simulink model "sysgen_oversample2x_2samples_per_clock"  (R2016b)
settings: Solver=VariableStepAuto  StartTime=0.0  StopTime=samples_per_channel*number_channels  RelTol=1e-3
PreLoadFcn:
  | setup
undefined symbols (not defined in the file or in its folder): j
libraries: xbsIndex_r4 x355, dspsigops x2, hdlsllib x2
(part 2 of 3)

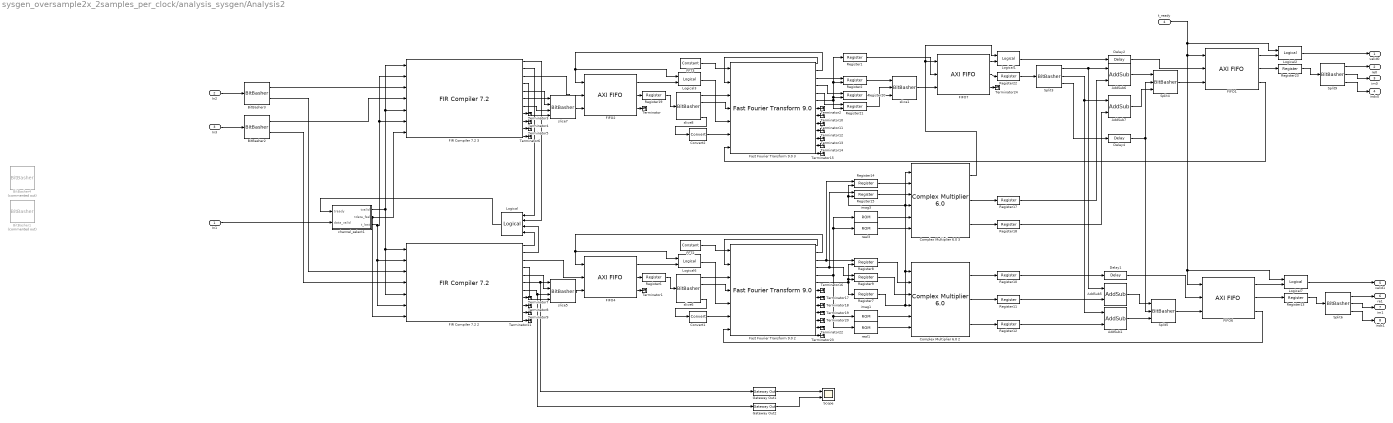
== system sysgen_oversample2x_2samples_per_clock/analysis_sysgen/Analysis2 ==
  In1 : Inport
  In2 : Inport  Port=2
  In3 : Inport  Port=3
  t_ready : Inport  Port=4
  AddSub{1,5..7} (4 alike) : xbsIndex_r4/AddSub  mode=Addition  use_carryin=off  use_carryout=off  en=off  latency=2  precision=Full  arith_type="Signed  (2's comp)"  n_bits=22  bin_pt=16  quantization=Truncate  overflow=Wrap  use_behavioral_HDL=on  hw_selection=Fabric  pipelined=off  dbl_ovrd=off  block_type=addsub
  BitBasher1 : xbsIndex_r4/BitBasher  Commented=on  bitexpr=|  display_expr=off  sr_1=lo  arith_type1="Signed  (2's comp)"  bin_pt1=15  sr_2=hi  arith_type2="Signed  (2's comp)"  bin_pt2=15  sr_3=hi  arith_type3=Unsigned  bin_pt3=0  sr_4=4  arith_type4=Unsigned  bin_pt4=0  dbl_ovrd=off  block_type=bitbasher
      | lo = {in[15:0]}
      | hi = {in[31:16]}
  BitBasher2 : xbsIndex_r4/BitBasher  bitexpr=|  display_expr=off  sr_1=hi  arith_type1="Signed  (2's comp)"  bin_pt1=15  sr_2=lo  arith_type2="Signed  (2's comp)"  bin_pt2=15  sr_3=hi  arith_type3=Unsigned  bin_pt3=0  sr_4=4  arith_type4=Unsigned  bin_pt4=0  dbl_ovrd=off  block_type=bitbasher
      | hi = {in[31:16]}
      | lo = {in[15:0]}
  BitBasher3 : xbsIndex_r4/BitBasher  bitexpr=|  display_expr=off  sr_1=hi  arith_type1="Signed  (2's comp)"  bin_pt1=15  sr_2=lo  arith_type2="Signed  (2's comp)"  bin_pt2=15  sr_3=hi  arith_type3=Unsigned  bin_pt3=0  sr_4=4  arith_type4=Unsigned  bin_pt4=0  dbl_ovrd=off  block_type=bitbasher
      | hi = {in[31:16]}
      | lo = {in[15:0]}
  BitBasher4 : xbsIndex_r4/BitBasher  Commented=on  bitexpr=|  display_expr=off  sr_1=lo  arith_type1="Signed  (2's comp)"  bin_pt1=15  sr_2=hi  arith_type2="Signed  (2's comp)"  bin_pt2=15  sr_3=hi  arith_type3=Unsigned  bin_pt3=0  sr_4=4  arith_type4=Unsigned  bin_pt4=0  dbl_ovrd=off  block_type=bitbasher
      | lo = {in[15:0]}
      | hi = {in[31:16]}
  Complex Multiplier 6.0 2 : xbsIndex_r4/Complex Multiplier 6.0   hasatlast=off  hasatuser=off  atuserwidth=1  hasbtlast=off  hasbtuser=off  btuserwidth=1  multtype=Use_Mults  optimizegoal=Resources  flowcontrol=NonBlocking  outputwidth=24  roundmode=Truncate  hasctrltlast=off  hasctrltuser=off  ctrltuserwidth=1  outtlastbehv=Null  latencyconfig=Automatic  minimumlatency=37  aclken=off  aresetn=off  trim_axipin_name=on  simulation_type=hybrid_sim  simulation_model=sysgen:cmpy_v6_0  data_path_portlist={ 's_axis_a_tdata_real', 's_axis_a_tdata_imag', 's_axis_b_tdata_real', 's_axis_b_tdata_imag', 's_axis_ctrl_tdata_rounding_bit', 'm_axis_dout_tdata_real', 'm_axis_dout_tdata_imag' }  aportwidth=63  bportwidth=63  ip_name=Complex Multiplier  ip_version=6.0  dsptool_ready=true  ipcore_usecache=true  ipcore_useipmodelcache=true  ipcore_verbose=false  ipcore_latency_parameter='minimumlatency'  wrapper_available=true  port_translation_map={ 'aclken' => 'en', 'aresetn' => 'rst'}  block_type=cmpy_v6_0
  Complex Multiplier 6.0 3 : xbsIndex_r4/Complex Multiplier 6.0   hasatlast=off  hasatuser=off  atuserwidth=1  hasbtlast=off  hasbtuser=off  btuserwidth=1  multtype=Use_Mults  optimizegoal=Resources  flowcontrol=NonBlocking  outputwidth=24  roundmode=Truncate  hasctrltlast=off  hasctrltuser=off  ctrltuserwidth=1  outtlastbehv=Null  latencyconfig=Automatic  minimumlatency=37  aclken=off  aresetn=off  trim_axipin_name=on  simulation_type=hybrid_sim  simulation_model=sysgen:cmpy_v6_0  data_path_portlist={ 's_axis_a_tdata_real', 's_axis_a_tdata_imag', 's_axis_b_tdata_real', 's_axis_b_tdata_imag', 's_axis_ctrl_tdata_rounding_bit', 'm_axis_dout_tdata_real', 'm_axis_dout_tdata_imag' }  aportwidth=63  bportwidth=63  ip_name=Complex Multiplier  ip_version=6.0  dsptool_ready=true  ipcore_usecache=true  ipcore_useipmodelcache=true  ipcore_verbose=false  ipcore_latency_parameter='minimumlatency'  wrapper_available=true  port_translation_map={ 'aclken' => 'en', 'aresetn' => 'rst'}  block_type=cmpy_v6_0
  Convert1 : xbsIndex_r4/Convert  gui_display_data_type=Boolean  arith_type=Boolean  n_bits=16  bin_pt=15  float_type=Single  exp_bits=8  fraction_bits=24  quantization=Truncate  overflow=Flag as error  en=off  latency=0  pipeline=off  dbl_ovrd=off  block_type=convert
  Convert2 : xbsIndex_r4/Convert  gui_display_data_type=Boolean  arith_type=Boolean  n_bits=16  bin_pt=15  float_type=Single  exp_bits=8  fraction_bits=24  quantization=Truncate  overflow=Flag as error  en=off  latency=0  pipeline=off  dbl_ovrd=off  block_type=convert
  Delay1 : xbsIndex_r4/Delay  rst=off  infoeditControl=Selection of Reset will increase slice count due to use of real FFs and instead of SRLs  en=off  latency=2  reg_retiming=on  dbl_ovrd=off  block_type=delay
  Delay2 : xbsIndex_r4/Delay  rst=off  infoeditControl=Selection of Reset will increase slice count due to use of real FFs and instead of SRLs  en=off  latency=2  reg_retiming=on  dbl_ovrd=off  block_type=delay
  Delay4 : xbsIndex_r4/Delay  rst=off  infoeditControl=Selection of Reset will increase slice count due to use of real FFs and instead of SRLs  en=off  latency=2  reg_retiming=on  dbl_ovrd=off  block_type=delay
  FFT2 : xbsIndex_r4/Constant  const=1  gui_display_data_type=Fixed-point  arith_type=Unsigned  n_bits=1  bin_pt=0  preci_type=Single  exp_width=8  frac_width=24  explicit_period=off  period=1  equ=P=C  opselect=C  inp2=PCIN>>17  opr=+  inp1=P  carry=CIN  dbl_ovrd=off  block_type=constant
  FFT3 : xbsIndex_r4/Constant  const=1  gui_display_data_type=Fixed-point  arith_type=Unsigned  n_bits=1  bin_pt=0  preci_type=Single  exp_width=8  frac_width=24  explicit_period=off  period=1  equ=P=C  opselect=C  inp2=PCIN>>17  opr=+  inp1=P  carry=CIN  dbl_ovrd=off  block_type=constant
  FIFO{1..2,4,6} (4 alike) : xbsIndex_r4/AXI FIFO  input_depth_axis=16  actual_fifo_depth_label=18  enable_tdata=on  enable_tdest=off  enable_tstrb=off  enable_tready=on  enable_tid=off  enable_tuser=off  enable_tkeep=off  enable_tlast=off  has_aresetn=off  enable_data_counts_axis=off  fifo_implementation_type_axis=Common Clock Distributed RAM  trim_axipin_name=on  programmable_full_type_axis=Full  full_threshold_assert_value_axis=0  programmable_empty_type_axis=Empty  empty_threshold_assert_value_axis=1022  underflow_flag_axi=0  underflow_sense_axi=Active High  overflow_flag_axi=0  overflow_sense_axi=Active High  block_type=axi_fifo
  FIFO7 : xbsIndex_r4/AXI FIFO  input_depth_axis=32  actual_fifo_depth_label=34  enable_tdata=on  enable_tdest=off  enable_tstrb=off  enable_tready=on  enable_tid=off  enable_tuser=off  enable_tkeep=off  enable_tlast=off  has_aresetn=off  enable_data_counts_axis=off  fifo_implementation_type_axis=Common Clock Distributed RAM  trim_axipin_name=on  programmable_full_type_axis=Full  full_threshold_assert_value_axis=0  programmable_empty_type_axis=Empty  empty_threshold_assert_value_axis=1022  underflow_flag_axi=0  underflow_sense_axi=Active High  overflow_flag_axi=0  overflow_sense_axi=Active High  block_type=axi_fifo
  FIR Compiler 7.2 2 : xbsIndex_r4/FIR Compiler 7.2   coefficientvector=analysis_coefficients2  coefficient_sets=8  coefficient_reload=off  filter_type=Single_Rate  rate_change_type=Integer  interpolation_rate=1  decimation_rate=1  zero_pack_factor=1  channel_sequence=Basic  number_channels=8  pattern_list='P4-0,P4-1,P4-2,P4-3,P4-4'  number_paths=2  ratespecification=Output_Sample_Period  sampleperiod=1.00000000  hardwareoversamplingrate=1  coefficient_sign=Signed  quantization=Quantize_Only  coefficient_width=25  bestprecision=on  coefficient_fractional_bits=28  coefficient_structure=Inferred  output_rounding_mode=Convergent_Rounding_to_Even  output_width=19  filter_architecture=Systolic_Multiply_Accumulate  optimization_goal=Area  optimization_list='None'  data_buffer_type=Automatic  coefficient_buffer_type=Automatic  input_buffer_type=Automatic  output_buffer_type=Automatic  preference_for_other_storage=Automatic  multi_column_support=Automatic  columnconfig='16'  inter_column_pipe_length=4  data_has_tlast=Vector_Framing  m_data_has_tready=off  s_data_has_fifo=off  s_data_has_tuser=Not_Required  m_data_has_tuser=Chan_ID_Field  s_config_sync_mode=On_Vector  s_config_method=By_Channel  num_reload_slots=1  has_aclken=off  has_aresetn=off  infoeditControl=ARESETn must be asserted for a minimum of 2 cycles  reset_data_vector=on  trim_axipin_name=on  simulation_type=hybrid_sim  simulation_model=sysgen:xfirv7_2_cmodel  data_path_portlist={ 's_axis_data_tdata', 'm_axis_data_tdata' }  passband_min=0.0  passband_max=0.5  stopband_min=0.5  stopband_max=1.0  filter_selection=1  gui_behaviour='Sysgen_GUI'  data_sign=Signed  data_width=16  data_fractional_bits=0  data_tuser_width=1  wrapper_available=true  ip_wrap_arbitrary_binary_point=true  ip_name=FIR Compiler  ip_version=7.2  dsptool_ready=true  ipcore_usecache=true  ipcore_useipmodelcache=true  port_translation_map={ 'aclken' => 'en', 'aresetn' => 'rst' }  run_core_at_system_period=true  ipcore_xco_need_fpga_part=true  block_type=fir_compiler_v7_2
      settings: infoedit=Maximum Possible : Maximizes oversampling rate. Abstracted input handshake (no s_data_tvalid) and automatic rate propagation.<br>Hardware Oversampling Rate : Specifies oversampling rate relative to the input sample period. Abstracted input handshake (no s_data_tvalid) and automatic rate propagation.<br>Input/Output Sample Period : Specifies absolute oversampling rate. No input handshake abstraction (exposes s_data_tvalid) and no rate propagation.
  FIR Compiler 7.2 3 : xbsIndex_r4/FIR Compiler 7.2   coefficientvector=analysis_coefficients1  coefficient_sets=8  coefficient_reload=off  filter_type=Single_Rate  rate_change_type=Integer  interpolation_rate=1  decimation_rate=1  zero_pack_factor=1  channel_sequence=Basic  number_channels=8  pattern_list='P4-0,P4-1,P4-2,P4-3,P4-4'  number_paths=2  ratespecification=Output_Sample_Period  sampleperiod=1.00000000  hardwareoversamplingrate=1  coefficient_sign=Signed  quantization=Quantize_Only  coefficient_width=25  bestprecision=on  coefficient_fractional_bits=28  coefficient_structure=Inferred  output_rounding_mode=Convergent_Rounding_to_Even  output_width=19  filter_architecture=Systolic_Multiply_Accumulate  optimization_goal=Area  optimization_list='None'  data_buffer_type=Automatic  coefficient_buffer_type=Automatic  input_buffer_type=Automatic  output_buffer_type=Automatic  preference_for_other_storage=Automatic  multi_column_support=Automatic  columnconfig='16'  inter_column_pipe_length=4  data_has_tlast=Vector_Framing  m_data_has_tready=off  s_data_has_fifo=off  s_data_has_tuser=Not_Required  m_data_has_tuser=Chan_ID_Field  s_config_sync_mode=On_Vector  s_config_method=By_Channel  num_reload_slots=1  has_aclken=off  has_aresetn=off  infoeditControl=ARESETn must be asserted for a minimum of 2 cycles  reset_data_vector=on  trim_axipin_name=on  simulation_type=hybrid_sim  simulation_model=sysgen:xfirv7_2_cmodel  data_path_portlist={ 's_axis_data_tdata', 'm_axis_data_tdata' }  passband_min=0.0  passband_max=0.5  stopband_min=0.5  stopband_max=1.0  filter_selection=1  gui_behaviour='Sysgen_GUI'  data_sign=Signed  data_width=16  data_fractional_bits=0  data_tuser_width=1  wrapper_available=true  ip_wrap_arbitrary_binary_point=true  ip_name=FIR Compiler  ip_version=7.2  dsptool_ready=true  ipcore_usecache=true  ipcore_useipmodelcache=true  port_translation_map={ 'aclken' => 'en', 'aresetn' => 'rst' }  run_core_at_system_period=true  ipcore_xco_need_fpga_part=true  block_type=fir_compiler_v7_2
      settings: infoedit=Maximum Possible : Maximizes oversampling rate. Abstracted input handshake (no s_data_tvalid) and automatic rate propagation.<br>Hardware Oversampling Rate : Specifies oversampling rate relative to the input sample period. Abstracted input handshake (no s_data_tvalid) and automatic rate propagation.<br>Input/Output Sample Period : Specifies absolute oversampling rate. No input handshake abstraction (exposes s_data_tvalid) and no rate propagation.
  Fast Fourier Transform 9.0 2 : xbsIndex_r4/Fast Fourier Transform 9.0   transform_length=8  target_clock_frequency=307  target_data_throughput=50  implementation_options=pipelined_streaming_io  run_time_configurable_transform_length=off  phase_factor_width=17  scaling_options=unscaled  rounding_modes=convergent_rounding  aclken=off  aresetn=off  output_ordering=natural_order  cyclic_prefix_insertion=off  throttle_scheme=nonrealtime  xk_index=on  ovflo=off  trim_axipin_name=on  memory_options_data=block_ram  memory_options_phase_factors=block_ram  number_of_stages_using_block_ram_for_data_and_phase_factors=0  memory_options_reorder=block_ram  memory_options_hybrid=off  complex_mult_type=use_mults_resources  butterfly_type=use_xtremedsp_slices  simulation_type=hybrid_sim  simulation_model=sysgen:xfftv9_cmodel  data_path_portlist={ 's_axis_data_tdata', 'm_axis_data_tdata', 'm_axis_status_tdata', 'event_fft_overflow' }  channels=1  input_ordering=natural_order  input_width=16  ip_name=Fast Fourier Transform  ip_version=9.0  dsptool_ready=true  ipcore_usecache=true  ipcore_useipmodelcache=true  wrapper_available=true  port_translation_map={ 'aclken' => 'en', 'aresetn' => 'rst'}  data_format=fixed_point  block_type=xfft_v9_0
  Fast Fourier Transform 9.0 3 : xbsIndex_r4/Fast Fourier Transform 9.0   transform_length=8  target_clock_frequency=307  target_data_throughput=50  implementation_options=pipelined_streaming_io  run_time_configurable_transform_length=off  phase_factor_width=17  scaling_options=unscaled  rounding_modes=convergent_rounding  aclken=off  aresetn=off  output_ordering=natural_order  cyclic_prefix_insertion=off  throttle_scheme=nonrealtime  xk_index=on  ovflo=off  trim_axipin_name=on  memory_options_data=block_ram  memory_options_phase_factors=block_ram  number_of_stages_using_block_ram_for_data_and_phase_factors=0  memory_options_reorder=block_ram  memory_options_hybrid=off  complex_mult_type=use_mults_resources  butterfly_type=use_xtremedsp_slices  simulation_type=hybrid_sim  simulation_model=sysgen:xfftv9_cmodel  data_path_portlist={ 's_axis_data_tdata', 'm_axis_data_tdata', 'm_axis_status_tdata', 'event_fft_overflow' }  channels=1  input_ordering=natural_order  input_width=16  ip_name=Fast Fourier Transform  ip_version=9.0  dsptool_ready=true  ipcore_usecache=true  ipcore_useipmodelcache=true  wrapper_available=true  port_translation_map={ 'aclken' => 'en', 'aresetn' => 'rst'}  data_format=fixed_point  block_type=xfft_v9_0
  Gateway Out1 : xbsIndex_r4/Gateway Out  inherit_from_input=off  hdl_port=off  rows=1  columns=1  UseAsDAC=off  DACChannel='1'  interface=None  automatic_assignment=on  address_offset=hex2dec('00')  intf_name=''  intf_description=''  timing_constraint=None  locs_specified=off  LOCs={}  io_standard={}  block_type=gatewayout
  Gateway Out2 : xbsIndex_r4/Gateway Out  inherit_from_input=off  hdl_port=off  rows=1  columns=1  UseAsDAC=off  DACChannel='1'  interface=None  automatic_assignment=on  address_offset=hex2dec('00')  intf_name=''  intf_description=''  timing_constraint=None  locs_specified=off  LOCs={}  io_standard={}  block_type=gatewayout
  Logical : xbsIndex_r4/Logical  logical_function=AND  inputs=4  en=off  latency=1  precision=Full  arith_type=Unsigned  n_bits=16  bin_pt=0  align_bp=on  dbl_ovrd=off  block_type=logical
  Logical{1..3,6..7} (5 alike) : xbsIndex_r4/Logical  logical_function=AND  inputs=2  en=off  latency=1  precision=Full  arith_type=Unsigned  n_bits=16  bin_pt=0  align_bp=on  dbl_ovrd=off  block_type=logical
  Register{1,6..7,10..13,17..19,22..23} (12 alike) : xbsIndex_r4/Register  init=0  rst=off  en=off  dbl_ovrd=off  block_type=register
  Register{2,8..9,14..15,20..21} (7 alike) : xbsIndex_r4/Register  init=0  rst=off  en=on  dbl_ovrd=off  block_type=register
  Scope : Scope  NumInputPorts=2
  Split3 : xbsIndex_r4/BitBasher  bitexpr=|  display_expr=off  sr_1=im  arith_type1="Signed  (2's comp)"  bin_pt1=17  sr_2=re  arith_type2="Signed  (2's comp)"  bin_pt2=17  sr_3=indx  arith_type3=Unsigned  bin_pt3=0  sr_4=4  arith_type4=Unsigned  bin_pt4=0  dbl_ovrd=off  block_type=bitbasher
      | im={in[43:22]}
      | re={in[21:0]}
      | indx = {in[46:44]}
  Split4 : xbsIndex_r4/BitBasher  bitexpr=out = {9'b0, indx, im, re}  display_expr=off  sr_1=out  arith_type1="Signed  (2's comp)"  bin_pt1=0  sr_2=im  arith_type2="Signed  (2's comp)"  bin_pt2=18  sr_3=3  arith_type3=Unsigned  bin_pt3=0  sr_4=4  arith_type4=Unsigned  bin_pt4=0  dbl_ovrd=off  block_type=bitbasher
  Split5 : xbsIndex_r4/BitBasher  bitexpr=out = {9'b0, indx, im, re}  display_expr=off  sr_1=out  arith_type1="Signed  (2's comp)"  bin_pt1=0  sr_2=im  arith_type2="Signed  (2's comp)"  bin_pt2=18  sr_3=3  arith_type3=Unsigned  bin_pt3=0  sr_4=4  arith_type4=Unsigned  bin_pt4=0  dbl_ovrd=off  block_type=bitbasher
  Split6 : xbsIndex_r4/BitBasher  bitexpr=|  display_expr=off  sr_1=re  arith_type1="Signed  (2's comp)"  bin_pt1=16  sr_2=im  arith_type2="Signed  (2's comp)"  bin_pt2=16  sr_3=indx  arith_type3=Unsigned  bin_pt3=0  sr_4=4  arith_type4=Unsigned  bin_pt4=0  dbl_ovrd=off  block_type=bitbasher
      | re={in[17:0]}
      | im={in[43:26]}
      | indx ={in[52:54]}
  Split9 : xbsIndex_r4/BitBasher  bitexpr=|  display_expr=off  sr_1=re  arith_type1="Signed  (2's comp)"  bin_pt1=16  sr_2=im  arith_type2="Signed  (2's comp)"  bin_pt2=16  sr_3=indx  arith_type3=Unsigned  bin_pt3=0  sr_4=4  arith_type4=Unsigned  bin_pt4=0  dbl_ovrd=off  block_type=bitbasher
      | re={in[17:0]}
      | im={in[43:26]}
      | indx ={in[54:52]}
  Terminator{,1..24} (25 alike) : Terminator
  channel_select1 : Subsystem
  imag1 : xbsIndex_r4/ROM  depth=8  initVector=imag(exp(-j*2*pi*(8:15)/16))  distributed_mem=Block RAM  rst=off  init_reg=0  en=off  latency=1  gui_display_data_type=Fixed-point  arith_type="Signed  (2's comp)"  n_bits=18  bin_pt=16  preci_type=Single  exp_width=8  frac_width=24  optimize=Area  use_rpm=on  dbl_ovrd=off  block_type=sprom
  imag3 : xbsIndex_r4/ROM  depth=8  initVector=imag(exp(-j*2*pi*(0:7)/16))  distributed_mem=Block RAM  rst=off  init_reg=0  en=off  latency=1  gui_display_data_type=Fixed-point  arith_type="Signed  (2's comp)"  n_bits=18  bin_pt=16  preci_type=Single  exp_width=8  frac_width=24  optimize=Area  use_rpm=on  dbl_ovrd=off  block_type=sprom
  real1 : xbsIndex_r4/ROM  depth=8  initVector=real(exp(-j*2*pi*(8:15)/16))  distributed_mem=Block RAM  rst=off  init_reg=0  en=off  latency=1  gui_display_data_type=Fixed-point  arith_type="Signed  (2's comp)"  n_bits=18  bin_pt=16  preci_type=Single  exp_width=8  frac_width=24  optimize=Area  use_rpm=on  dbl_ovrd=off  block_type=sprom
  real3 : xbsIndex_r4/ROM  depth=8  initVector=real(exp(-j*2*pi*(0:7)/16))  distributed_mem=Block RAM  rst=off  init_reg=0  en=off  latency=1  gui_display_data_type=Fixed-point  arith_type="Signed  (2's comp)"  n_bits=18  bin_pt=16  preci_type=Single  exp_width=8  frac_width=24  optimize=Area  use_rpm=on  dbl_ovrd=off  block_type=sprom
  slice1 : xbsIndex_r4/BitBasher  bitexpr="out ={17'b0,  indx, im, re }"  display_expr=off  sr_1=out  arith_type1=Unsigned  bin_pt1=0  sr_2=2  arith_type2="Signed  (2's comp)"  bin_pt2=16  sr_3=3  arith_type3=Unsigned  bin_pt3=0  sr_4=4  arith_type4=Unsigned  bin_pt4=0  dbl_ovrd=off  block_type=bitbasher
  slice5 : xbsIndex_r4/BitBasher  bitexpr=out ={19'b0, tlast, indx, im[20:0], re[20:0] }  display_expr=off  sr_1=out  arith_type1=Unsigned  bin_pt1=0  sr_2=2  arith_type2="Signed  (2's comp)"  bin_pt2=16  sr_3=3  arith_type3=Unsigned  bin_pt3=0  sr_4=4  arith_type4=Unsigned  bin_pt4=0  dbl_ovrd=off  block_type=bitbasher
  slice6 : xbsIndex_r4/BitBasher  bitexpr=|  display_expr=off  sr_1=im_out  arith_type1="Signed  (2's comp)"  bin_pt1=17  sr_2=re_out  arith_type2="Signed  (2's comp)"  bin_pt2=17  sr_3=indx  arith_type3=Unsigned  bin_pt3=0  sr_4=tlast  arith_type4=Unsigned  bin_pt4=0  dbl_ovrd=off  block_type=bitbasher
      | im_out ={ in[39:22] }
      | re_out = { in[18:1] }
      | indx    = { in[44:42] } 
      | tlast     = { in[45] }
  slice7 : xbsIndex_r4/BitBasher  bitexpr=out ={19'b0, tlast, indx, im[20:0], re[20:0] }  display_expr=off  sr_1=out  arith_type1=Unsigned  bin_pt1=0  sr_2=2  arith_type2="Signed  (2's comp)"  bin_pt2=16  sr_3=3  arith_type3=Unsigned  bin_pt3=0  sr_4=4  arith_type4=Unsigned  bin_pt4=0  dbl_ovrd=off  block_type=bitbasher
  slice8 : xbsIndex_r4/BitBasher  bitexpr=|  display_expr=off  sr_1=im_out  arith_type1="Signed  (2's comp)"  bin_pt1=17  sr_2=re_out  arith_type2="Signed  (2's comp)"  bin_pt2=17  sr_3=indx  arith_type3=Unsigned  bin_pt3=0  sr_4=tlast  arith_type4=Unsigned  bin_pt4=0  dbl_ovrd=off  block_type=bitbasher
      | im_out ={ in[39:22] }
      | re_out = { in[18:1] }
      | indx    = { in[44:42] } 
      | tlast     = { in[45] }
  valid0 : Outport
  re0 : Outport  Port=2
  im0 : Outport  Port=3
  indx0 : Outport  Port=4
  valid1 : Outport  Port=5
  re1 : Outport  Port=6
  im1 : Outport  Port=7
  indx1 : Outport  Port=8
  wires:
  FIR Compiler 7.2 2/6 -> slice5/1, Gateway Out1/1
  slice6/1 -> Fast Fourier Transform 9.0 2/3
  Gateway Out2/1 -> Scope/2
  Gateway Out1/1 -> Scope/1
  Fast Fourier Transform 9.0 2/5 -> imag3/1, real3/1, imag1/1, real1/1
  FIFO2/1 -> Logical3/2
  FIFO7/3 -> Terminator24/1
  Fast Fourier Transform 9.0 2/13 -> Terminator23/1
  Fast Fourier Transform 9.0 2/12 -> Terminator22/1
  Fast Fourier Transform 9.0 2/11 -> Terminator20/1
  Fast Fourier Transform 9.0 2/10 -> Terminator19/1
  Fast Fourier Transform 9.0 2/9 -> Terminator18/1
  Fast Fourier Transform 9.0 2/8 -> Terminator17/1
  Fast Fourier Transform 9.0 2/7 -> Terminator16/1
  Fast Fourier Transform 9.0 3/13 -> Terminator15/1
  Fast Fourier Transform 9.0 3/12 -> Terminator14/1
  Fast Fourier Transform 9.0 3/11 -> Terminator13/1
  Fast Fourier Transform 9.0 3/10 -> Terminator12/1
  Fast Fourier Transform 9.0 3/9 -> Terminator11/1
  Fast Fourier Transform 9.0 3/8 -> Terminator10/1
  Fast Fourier Transform 9.0 3/7 -> Terminator2/1
  FIFO4/3 -> Terminator1/1
  FIFO2/3 -> Terminator/1
  Split3/3 -> Delay4/1
  FIFO1/3 -> Fast Fourier Transform 9.0 3/7
  FIFO6/3 -> Fast Fourier Transform 9.0 2/7
  FIFO1/2 -> Register23/1
  FIFO1/1 -> Logical2/2
  Split9/3 -> indx0/1
  Split9/2 -> im0/1
  Split9/1 -> re0/1
  Logical2/1 -> valid0/1
  Register23/1 -> Split9/1
  Delay2/1 -> FIFO1/2
  Split4/1 -> FIFO1/3
  AddSub7/1 -> Split4/3
  AddSub6/1 -> Split4/1
  Delay4/1 -> Split4/2, Split5/2
  Logical1/1 -> Delay2/1
  Register18/1 -> AddSub7/2
  Register17/1 -> AddSub6/2
  Split3/2 -> AddSub7/1, AddSub1/1
  Split3/1 -> AddSub6/1, AddSub5/1
  Register22/1 -> Split3/1
  FIFO7/1 -> Logical1/2
  FIFO7/2 -> Register22/1
  slice1/1 -> FIFO7/3
  Register1/1 -> FIFO7/2
  Register20/1 -> slice1/3
  Register21/1 -> slice1/2
  Register2/1 -> slice1/1
  Fast Fourier Transform 9.0 3/5 -> Register21/1
  Fast Fourier Transform 9.0 3/6 -> Register21/2, Register20/2, Register2/2, Register1/1
  Fast Fourier Transform 9.0 3/4 -> Register20/1
  Fast Fourier Transform 9.0 3/3 -> Register2/1
  BitBasher2/1 -> FIR Compiler 7.2 3/4
  BitBasher3/1 -> FIR Compiler 7.2 3/3
  channel_select1/3(t_last) -> FIR Compiler 7.2 2/2, FIR Compiler 7.2 2/6, FIR Compiler 7.2 3/6, FIR Compiler 7.2 3/2
  Convert2/1 -> Fast Fourier Transform 9.0 3/6
  Fast Fourier Transform 9.0 3/1 -> Fast Fourier Transform 9.0 3/2
  FFT3/1 -> Fast Fourier Transform 9.0 3/1
  slice8/4 -> Convert2/1
  Logical3/1 -> Fast Fourier Transform 9.0 3/5
  slice8/2 -> Fast Fourier Transform 9.0 3/4
  slice8/1 -> Fast Fourier Transform 9.0 3/3
  Register19/1 -> slice8/1
  FIFO2/2 -> Register19/1
  Fast Fourier Transform 9.0 3/2 -> Logical3/1, FIFO2/1
  FIR Compiler 7.2 2/11 -> Terminator21/1
  FIR Compiler 7.2 2/10 -> Terminator9/1
  FIR Compiler 7.2 2/9 -> Terminator8/1
  FIR Compiler 7.2 2/8 -> Terminator7/1
  FIR Compiler 7.2 3/11 -> Terminator6/1
  FIR Compiler 7.2 3/10 -> Terminator5/1
  FIR Compiler 7.2 3/9 -> Terminator4/1
  FIR Compiler 7.2 3/8 -> Terminator3/1
  FIR Compiler 7.2 3/3 -> FIFO2/2
  slice7/1 -> FIFO2/3
  FIR Compiler 7.2 3/4 -> slice7/4
  FIR Compiler 7.2 3/5 -> slice7/2
  FIR Compiler 7.2 3/7 -> slice7/3
  FIR Compiler 7.2 3/6 -> slice7/1
  FIR Compiler 7.2 3/2 -> Logical/1
  FIR Compiler 7.2 3/1 -> Logical/2
  FIR Compiler 7.2 2/2 -> Logical/3
  FIR Compiler 7.2 2/1 -> Logical/4
  Complex Multiplier 6.0 3/3 -> Register18/1
  Complex Multiplier 6.0 3/2 -> Register17/1
  Complex Multiplier 6.0 3/1 -> FIFO7/1, Logical1/1
  Register14/1 -> Complex Multiplier 6.0 3/2
  Register15/1 -> Complex Multiplier 6.0 3/3
  real3/1 -> Complex Multiplier 6.0 3/6
  imag3/1 -> Complex Multiplier 6.0 3/5
  Split6/3 -> indx1/1
  Split6/2 -> im1/1
  Split6/1 -> re1/1
  Logical7/1 -> valid1/1
  Register13/1 -> Split6/1
  FIFO6/2 -> Register13/1
  FIFO6/1 -> Logical7/2
  Delay1/1 -> FIFO6/2
  Split5/1 -> FIFO6/3
  AddSub1/1 -> Split5/3
  AddSub5/1 -> Split5/1
  Register10/1 -> Delay1/1
  Register11/1 -> AddSub5/2
  Register12/1 -> AddSub1/2
  Complex Multiplier 6.0 2/1 -> Register10/1
  Complex Multiplier 6.0 2/2 -> Register11/1
  Complex Multiplier 6.0 2/3 -> Register12/1
  Register7/1 -> Complex Multiplier 6.0 2/4, Complex Multiplier 6.0 2/1, Complex Multiplier 6.0 3/1, Complex Multiplier 6.0 3/4, Register15/2, Register14/2
  Register8/1 -> Complex Multiplier 6.0 2/2
  Register9/1 -> Complex Multiplier 6.0 2/3
  real1/1 -> Complex Multiplier 6.0 2/6
  imag1/1 -> Complex Multiplier 6.0 2/5
  Fast Fourier Transform 9.0 2/6 -> Register7/1, Register9/2, Register8/2
  Fast Fourier Transform 9.0 2/4 -> Register9/1, Register15/1
  Fast Fourier Transform 9.0 2/3 -> Register8/1, Register14/1
  Convert1/1 -> Fast Fourier Transform 9.0 2/6
  Fast Fourier Transform 9.0 2/1 -> Fast Fourier Transform 9.0 2/2
  FFT2/1 -> Fast Fourier Transform 9.0 2/1
  slice6/4 -> Convert1/1
  FIR Compiler 7.2 2/4 -> slice5/4
  Logical6/1 -> Fast Fourier Transform 9.0 2/5
  slice6/2 -> Fast Fourier Transform 9.0 2/4
  Register6/1 -> slice6/1
  FIFO4/2 -> Register6/1
  Fast Fourier Transform 9.0 2/2 -> FIFO4/1, Logical6/1
  FIFO4/1 -> Logical6/2
  FIR Compiler 7.2 2/3 -> FIFO4/2
  slice5/1 -> FIFO4/3
  FIR Compiler 7.2 2/5 -> slice5/2
  FIR Compiler 7.2 2/7 -> slice5/3, Gateway Out2/1
  Logical/1 -> channel_select1/1(tready)
  In1/1 -> channel_select1/2(data_valid)
  BitBasher2/2 -> FIR Compiler 7.2 2/4
  In3/1 -> BitBasher2/1
  BitBasher3/2 -> FIR Compiler 7.2 2/3
  In2/1 -> BitBasher3/1
  channel_select1/1(tvalid) -> FIR Compiler 7.2 2/1, FIR Compiler 7.2 2/5, FIR Compiler 7.2 3/1, FIR Compiler 7.2 3/5
  channel_select1/2(tdata_fsel) -> FIR Compiler 7.2 3/7, FIR Compiler 7.2 2/7
  t_ready/1 -> FIFO6/1, Logical7/1, FIFO1/1, Logical2/1

== system sysgen_oversample2x_2samples_per_clock/analysis_sysgen/Enabled Subsystem ==
  In1 : Inport
  Enable : EnablePort
  Buffer : Buffer  N=8  TreatMby1Signals=One channel  OutputFrames=off
  Out1 : Outport
  wires:
  In1/1 -> Buffer/1
  Buffer/1 -> Out1/1

== system sysgen_oversample2x_2samples_per_clock/analysis_sysgen/Enabled Subsystem2 ==
  In1 : Inport
  Enable : EnablePort
  Buffer : Buffer  N=8  TreatMby1Signals=One channel  OutputFrames=off
  Out1 : Outport
  wires:
  Buffer/1 -> Out1/1
  In1/1 -> Buffer/1

== system sysgen_oversample2x_2samples_per_clock/analysis_sysgen/Enabled Subsystem3 ==
  In1 : Inport
  Enable : EnablePort
  Buffer : Buffer  N=8  TreatMby1Signals=One channel  OutputFrames=off
  Out1 : Outport
  wires:
  In1/1 -> Buffer/1
  Buffer/1 -> Out1/1

== system sysgen_oversample2x_2samples_per_clock/analysis_sysgen/Enabled Subsystem4 ==
  In1 : Inport
  Enable : EnablePort
  Buffer : Buffer  N=8  TreatMby1Signals=One channel  OutputFrames=off
  Out1 : Outport
  wires:
  In1/1 -> Buffer/1
  Buffer/1 -> Out1/1

== system sysgen_oversample2x_2samples_per_clock/analysis_sysgen/Pre-Analysis0 ==
  valid : Inport
  im : Inport  Port=2
  re : Inport  Port=3
  Delay : xbsIndex_r4/Delay  rst=off  infoeditControl=Selection of Reset will increase slice count due to use of real FFs and instead of SRLs  en=off  latency=7  reg_retiming=on  dbl_ovrd=off  block_type=delay
  Delay1 : xbsIndex_r4/Delay  rst=off  infoeditControl=Selection of Reset will increase slice count due to use of real FFs and instead of SRLs  en=off  latency=7  reg_retiming=on  dbl_ovrd=off  block_type=delay
  Delay2 : xbsIndex_r4/Delay  rst=off  infoeditControl=Selection of Reset will increase slice count due to use of real FFs and instead of SRLs  en=off  latency=7  reg_retiming=on  dbl_ovrd=off  block_type=delay
  valid0 : Outport
  im0 : Outport  Port=2
  reo : Outport  Port=3
  wires:
  valid/1 -> Delay/1
  im/1 -> Delay1/1
  re/1 -> Delay2/1
  Delay/1 -> valid0/1
  Delay1/1 -> im0/1
  Delay2/1 -> reo/1

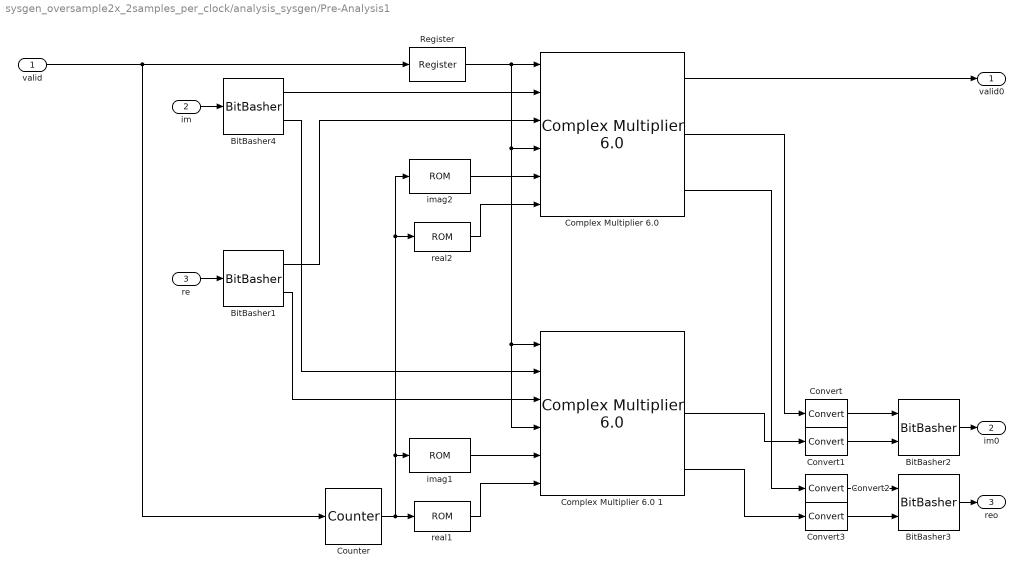
== system sysgen_oversample2x_2samples_per_clock/analysis_sysgen/Pre-Analysis1 ==
  valid : Inport
  im : Inport  Port=2
  re : Inport  Port=3
  BitBasher1 : xbsIndex_r4/BitBasher  bitexpr=|  display_expr=off  sr_1=hi  arith_type1="Signed  (2's comp)"  bin_pt1=15  sr_2=lo  arith_type2="Signed  (2's comp)"  bin_pt2=15  sr_3=hi  arith_type3=Unsigned  bin_pt3=0  sr_4=4  arith_type4=Unsigned  bin_pt4=0  dbl_ovrd=off  block_type=bitbasher
      | hi = {in[31:16]}
      | lo = {in[15:0]}
  BitBasher2 : xbsIndex_r4/BitBasher  bitexpr=out = {hi, lo}  display_expr=off  sr_1=out  arith_type1=Unsigned  bin_pt1=0  sr_2=hi  arith_type2="Signed  (2's comp)"  bin_pt2=15  sr_3=hi  arith_type3=Unsigned  bin_pt3=0  sr_4=4  arith_type4=Unsigned  bin_pt4=0  dbl_ovrd=off  block_type=bitbasher
  BitBasher3 : xbsIndex_r4/BitBasher  bitexpr=out = {hi, lo}  display_expr=off  sr_1=out  arith_type1=Unsigned  bin_pt1=0  sr_2=hi  arith_type2="Signed  (2's comp)"  bin_pt2=15  sr_3=hi  arith_type3=Unsigned  bin_pt3=0  sr_4=4  arith_type4=Unsigned  bin_pt4=0  dbl_ovrd=off  block_type=bitbasher
  BitBasher4 : xbsIndex_r4/BitBasher  bitexpr=|  display_expr=off  sr_1=hi  arith_type1="Signed  (2's comp)"  bin_pt1=15  sr_2=lo  arith_type2="Signed  (2's comp)"  bin_pt2=15  sr_3=hi  arith_type3=Unsigned  bin_pt3=0  sr_4=4  arith_type4=Unsigned  bin_pt4=0  dbl_ovrd=off  block_type=bitbasher
      | hi = {in[31:16]}
      | lo = {in[15:0]}
  "Complex Multiplier 6.0 " : xbsIndex_r4/Complex Multiplier 6.0   hasatlast=off  hasatuser=off  atuserwidth=1  hasbtlast=off  hasbtuser=off  btuserwidth=1  multtype=Use_Mults  optimizegoal=Resources  flowcontrol=NonBlocking  outputwidth=19  roundmode=Truncate  hasctrltlast=off  hasctrltuser=off  ctrltuserwidth=1  outtlastbehv=Null  latencyconfig=Automatic  minimumlatency=37  aclken=off  aresetn=off  trim_axipin_name=on  simulation_type=hybrid_sim  simulation_model=sysgen:cmpy_v6_0  data_path_portlist={ 's_axis_a_tdata_real', 's_axis_a_tdata_imag', 's_axis_b_tdata_real', 's_axis_b_tdata_imag', 's_axis_ctrl_tdata_rounding_bit', 'm_axis_dout_tdata_real', 'm_axis_dout_tdata_imag' }  aportwidth=63  bportwidth=63  ip_name=Complex Multiplier  ip_version=6.0  dsptool_ready=true  ipcore_usecache=true  ipcore_useipmodelcache=true  ipcore_verbose=false  ipcore_latency_parameter='minimumlatency'  wrapper_available=true  port_translation_map={ 'aclken' => 'en', 'aresetn' => 'rst'}  block_type=cmpy_v6_0
  Complex Multiplier 6.0 1 : xbsIndex_r4/Complex Multiplier 6.0   hasatlast=off  hasatuser=off  atuserwidth=1  hasbtlast=off  hasbtuser=off  btuserwidth=1  multtype=Use_Mults  optimizegoal=Resources  flowcontrol=NonBlocking  outputwidth=19  roundmode=Truncate  hasctrltlast=off  hasctrltuser=off  ctrltuserwidth=1  outtlastbehv=Null  latencyconfig=Automatic  minimumlatency=37  aclken=off  aresetn=off  trim_axipin_name=on  simulation_type=hybrid_sim  simulation_model=sysgen:cmpy_v6_0  data_path_portlist={ 's_axis_a_tdata_real', 's_axis_a_tdata_imag', 's_axis_b_tdata_real', 's_axis_b_tdata_imag', 's_axis_ctrl_tdata_rounding_bit', 'm_axis_dout_tdata_real', 'm_axis_dout_tdata_imag' }  aportwidth=63  bportwidth=63  ip_name=Complex Multiplier  ip_version=6.0  dsptool_ready=true  ipcore_usecache=true  ipcore_useipmodelcache=true  ipcore_verbose=false  ipcore_latency_parameter='minimumlatency'  wrapper_available=true  port_translation_map={ 'aclken' => 'en', 'aresetn' => 'rst'}  block_type=cmpy_v6_0
  Convert{,1..3} (4 alike) : xbsIndex_r4/Convert  gui_display_data_type=Fixed-point  arith_type="Signed  (2's comp)"  n_bits=16  bin_pt=15  float_type=Single  exp_bits=8  fraction_bits=24  quantization=Truncate  overflow=Flag as error  en=off  latency=0  pipeline=off  dbl_ovrd=off  block_type=convert
  Counter : xbsIndex_r4/Counter  cnt_type=Free Running  cnt_to=Inf  operation=Up  start_count=0  cnt_by_val=1  arith_type=Unsigned  n_bits=4  bin_pt=0  load_pin=off  rst=off  en=on  explicit_period=on  period=2  use_behavioral_HDL=off  implementation=Fabric  dbl_ovrd=off  block_type=counter
  Register : xbsIndex_r4/Register  init=0  rst=off  en=off  dbl_ovrd=off  block_type=register
  imag1 : xbsIndex_r4/ROM  depth=16  initVector=imag(exp(-j*2*pi*(1:2:31)/32))  distributed_mem=Block RAM  rst=off  init_reg=0  en=off  latency=1  gui_display_data_type=Fixed-point  arith_type="Signed  (2's comp)"  n_bits=18  bin_pt=16  preci_type=Single  exp_width=8  frac_width=24  optimize=Area  use_rpm=on  dbl_ovrd=off  block_type=sprom
  imag2 : xbsIndex_r4/ROM  depth=16  initVector=imag(exp(-j*2*pi*(0:2:31)/32))  distributed_mem=Block RAM  rst=off  init_reg=0  en=off  latency=1  gui_display_data_type=Fixed-point  arith_type="Signed  (2's comp)"  n_bits=18  bin_pt=16  preci_type=Single  exp_width=8  frac_width=24  optimize=Area  use_rpm=on  dbl_ovrd=off  block_type=sprom
  real1 : xbsIndex_r4/ROM  depth=16  initVector=real(exp(-j*2*pi*(1:2:31)/32))  distributed_mem=Block RAM  rst=off  init_reg=0  en=off  latency=1  gui_display_data_type=Fixed-point  arith_type="Signed  (2's comp)"  n_bits=18  bin_pt=16  preci_type=Single  exp_width=8  frac_width=24  optimize=Area  use_rpm=on  dbl_ovrd=off  block_type=sprom
  real2 : xbsIndex_r4/ROM  depth=16  initVector=real(exp(-j*2*pi*(0:2:31)/32))  distributed_mem=Block RAM  rst=off  init_reg=0  en=off  latency=1  gui_display_data_type=Fixed-point  arith_type="Signed  (2's comp)"  n_bits=18  bin_pt=16  preci_type=Single  exp_width=8  frac_width=24  optimize=Area  use_rpm=on  dbl_ovrd=off  block_type=sprom
  valid0 : Outport
  im0 : Outport  Port=2
  reo : Outport  Port=3
  wires:
  im/1 -> BitBasher4/1
  re/1 -> BitBasher1/1
  real2/1 -> "Complex Multiplier 6.0 "/6
  imag2/1 -> "Complex Multiplier 6.0 "/5
  BitBasher4/1 -> "Complex Multiplier 6.0 "/2
  real1/1 -> Complex Multiplier 6.0 1/6
  imag1/1 -> Complex Multiplier 6.0 1/5
  BitBasher4/2 -> Complex Multiplier 6.0 1/2
  BitBasher1/2 -> Complex Multiplier 6.0 1/3
  Counter/1 -> imag2/1, real2/1, imag1/1, real1/1
  BitBasher2/1 -> im0/1
  BitBasher3/1 -> reo/1
  valid/1 -> Register/1, Counter/1
  Convert/1 -> BitBasher2/1
  Convert2/1 -> BitBasher3/1
  Convert3/1 -> BitBasher3/2
  Register/1 -> "Complex Multiplier 6.0 "/4, Complex Multiplier 6.0 1/1, Complex Multiplier 6.0 1/4, "Complex Multiplier 6.0 "/1
  "Complex Multiplier 6.0 "/1 -> valid0/1
  Convert1/1 -> BitBasher2/2
  BitBasher1/1 -> "Complex Multiplier 6.0 "/3
  Complex Multiplier 6.0 1/2 -> Convert1/1
  Complex Multiplier 6.0 1/3 -> Convert3/1
  "Complex Multiplier 6.0 "/2 -> Convert/1
  "Complex Multiplier 6.0 "/3 -> Convert2/1

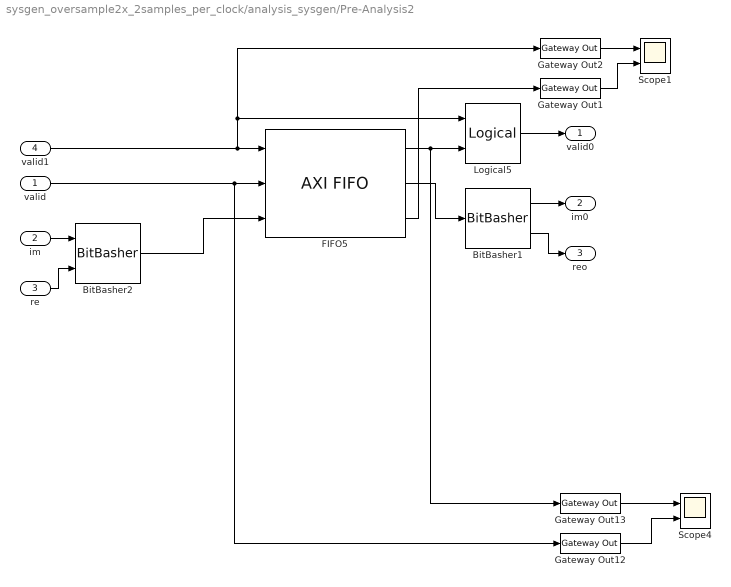
== system sysgen_oversample2x_2samples_per_clock/analysis_sysgen/Pre-Analysis2 ==
  valid : Inport
  im : Inport  Port=2
  re : Inport  Port=3
  valid1 : Inport  Port=4
  BitBasher1 : xbsIndex_r4/BitBasher  bitexpr=|  display_expr=off  sr_1=im  arith_type1=Unsigned  bin_pt1=0  sr_2=re  arith_type2=Unsigned  bin_pt2=0  sr_3=hi  arith_type3=Unsigned  bin_pt3=0  sr_4=4  arith_type4=Unsigned  bin_pt4=0  dbl_ovrd=off  block_type=bitbasher
      | im = {in[63:32]}
      | re = {in[31:0]}
  BitBasher2 : xbsIndex_r4/BitBasher  bitexpr=out = {im, re}  display_expr=off  sr_1=out  arith_type1=Unsigned  bin_pt1=0  sr_2=hi  arith_type2="Signed  (2's comp)"  bin_pt2=15  sr_3=hi  arith_type3=Unsigned  bin_pt3=0  sr_4=4  arith_type4=Unsigned  bin_pt4=0  dbl_ovrd=off  block_type=bitbasher
  FIFO5 : xbsIndex_r4/AXI FIFO  input_depth_axis=16  actual_fifo_depth_label=18  enable_tdata=on  enable_tdest=off  enable_tstrb=off  enable_tready=on  enable_tid=off  enable_tuser=off  enable_tkeep=off  enable_tlast=off  has_aresetn=off  enable_data_counts_axis=off  fifo_implementation_type_axis=Common Clock Distributed RAM  trim_axipin_name=on  programmable_full_type_axis=Full  full_threshold_assert_value_axis=0  programmable_empty_type_axis=Empty  empty_threshold_assert_value_axis=1022  underflow_flag_axi=0  underflow_sense_axi=Active High  overflow_flag_axi=0  overflow_sense_axi=Active High  block_type=axi_fifo
  Gateway Out{1..2,12..13} (4 alike) : xbsIndex_r4/Gateway Out  inherit_from_input=off  hdl_port=off  rows=1  columns=1  UseAsDAC=off  DACChannel='1'  interface=None  automatic_assignment=on  address_offset=hex2dec('00')  intf_name=''  intf_description=''  timing_constraint=None  locs_specified=off  LOCs={}  io_standard={}  block_type=gatewayout
  Logical5 : xbsIndex_r4/Logical  logical_function=AND  inputs=2  en=off  latency=0  precision=Full  arith_type=Unsigned  n_bits=16  bin_pt=0  align_bp=on  dbl_ovrd=off  block_type=logical
  Scope1 : Scope  NumInputPorts=2
  Scope4 : Scope  NumInputPorts=2
  valid0 : Outport
  im0 : Outport  Port=2
  reo : Outport  Port=3
  wires:
  Gateway Out12/1 -> Scope4/2
  Gateway Out13/1 -> Scope4/1
  FIFO5/2 -> BitBasher1/1
  BitBasher1/2 -> reo/1
  BitBasher1/1 -> im0/1
  Logical5/1 -> valid0/1
  FIFO5/1 -> Logical5/2, Gateway Out13/1
  BitBasher2/1 -> FIFO5/3
  re/1 -> BitBasher2/2
  im/1 -> BitBasher2/1
  valid/1 -> FIFO5/2, Gateway Out12/1
  FIFO5/3 -> Gateway Out1/1
  Gateway Out2/1 -> Scope1/1
  Gateway Out1/1 -> Scope1/2
  valid1/1 -> FIFO5/1, Gateway Out2/1, Logical5/1

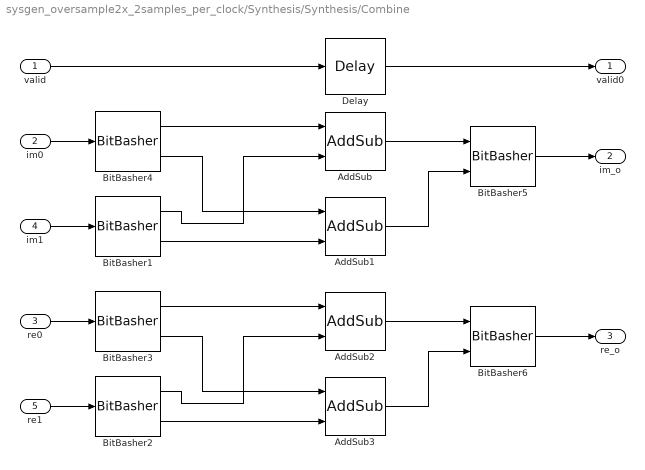
== system sysgen_oversample2x_2samples_per_clock/Synthesis/Synthesis/Combine ==
  valid : Inport
  im0 : Inport  Port=2
  re0 : Inport  Port=3
  im1 : Inport  Port=4
  re1 : Inport  Port=5
  AddSub{,1..3} (4 alike) : xbsIndex_r4/AddSub  mode=Subtraction  use_carryin=off  use_carryout=off  en=off  latency=2  precision=User Defined  arith_type="Signed  (2's comp)"  n_bits=16  bin_pt=15  quantization=Truncate  overflow=Saturate  use_behavioral_HDL=on  hw_selection=Fabric  pipelined=off  dbl_ovrd=off  block_type=addsub
  BitBasher1 : xbsIndex_r4/BitBasher  bitexpr=|  display_expr=off  sr_1=hi  arith_type1="Signed  (2's comp)"  bin_pt1=15  sr_2=lo  arith_type2="Signed  (2's comp)"  bin_pt2=15  sr_3=hi  arith_type3=Unsigned  bin_pt3=0  sr_4=4  arith_type4=Unsigned  bin_pt4=0  dbl_ovrd=off  block_type=bitbasher
      | hi = {in[31:16]}
      | lo = {in[15:0]}
  BitBasher2 : xbsIndex_r4/BitBasher  bitexpr=|  display_expr=off  sr_1=hi  arith_type1="Signed  (2's comp)"  bin_pt1=15  sr_2=lo  arith_type2="Signed  (2's comp)"  bin_pt2=15  sr_3=hi  arith_type3=Unsigned  bin_pt3=0  sr_4=4  arith_type4=Unsigned  bin_pt4=0  dbl_ovrd=off  block_type=bitbasher
      | hi = {in[31:16]}
      | lo = {in[15:0]}
  BitBasher3 : xbsIndex_r4/BitBasher  bitexpr=|  display_expr=off  sr_1=hi  arith_type1="Signed  (2's comp)"  bin_pt1=15  sr_2=lo  arith_type2="Signed  (2's comp)"  bin_pt2=15  sr_3=hi  arith_type3=Unsigned  bin_pt3=0  sr_4=4  arith_type4=Unsigned  bin_pt4=0  dbl_ovrd=off  block_type=bitbasher
      | hi = {in[31:16]}
      | lo = {in[15:0]}
  BitBasher4 : xbsIndex_r4/BitBasher  bitexpr=|  display_expr=off  sr_1=hi  arith_type1="Signed  (2's comp)"  bin_pt1=15  sr_2=lo  arith_type2="Signed  (2's comp)"  bin_pt2=15  sr_3=hi  arith_type3=Unsigned  bin_pt3=0  sr_4=4  arith_type4=Unsigned  bin_pt4=0  dbl_ovrd=off  block_type=bitbasher
      | hi = {in[31:16]}
      | lo = {in[15:0]}
  BitBasher5 : xbsIndex_r4/BitBasher  bitexpr=out = {hi, lo}  display_expr=off  sr_1=out  arith_type1=Unsigned  bin_pt1=0  sr_2=hi  arith_type2="Signed  (2's comp)"  bin_pt2=15  sr_3=hi  arith_type3=Unsigned  bin_pt3=0  sr_4=4  arith_type4=Unsigned  bin_pt4=0  dbl_ovrd=off  block_type=bitbasher
  BitBasher6 : xbsIndex_r4/BitBasher  bitexpr=out = {hi, lo}  display_expr=off  sr_1=out  arith_type1=Unsigned  bin_pt1=0  sr_2=hi  arith_type2="Signed  (2's comp)"  bin_pt2=15  sr_3=hi  arith_type3=Unsigned  bin_pt3=0  sr_4=4  arith_type4=Unsigned  bin_pt4=0  dbl_ovrd=off  block_type=bitbasher
  Delay : xbsIndex_r4/Delay  rst=off  infoeditControl=Selection of Reset will increase slice count due to use of real FFs and instead of SRLs  en=off  latency=2  reg_retiming=on  dbl_ovrd=off  block_type=delay
  valid0 : Outport
  im_o : Outport  Port=2
  re_o : Outport  Port=3
  wires:
  im1/1 -> BitBasher1/1
  im0/1 -> BitBasher4/1
  valid/1 -> Delay/1
  BitBasher4/1 -> AddSub/1
  BitBasher1/1 -> AddSub/2
  BitBasher4/2 -> AddSub1/1
  BitBasher1/2 -> AddSub1/2
  re1/1 -> BitBasher2/1
  re0/1 -> BitBasher3/1
  BitBasher3/1 -> AddSub2/1
  BitBasher2/1 -> AddSub2/2
  BitBasher3/2 -> AddSub3/1
  BitBasher2/2 -> AddSub3/2
  Delay/1 -> valid0/1
  AddSub/1 -> BitBasher5/1
  AddSub1/1 -> BitBasher5/2
  AddSub2/1 -> BitBasher6/1
  AddSub3/1 -> BitBasher6/2
  BitBasher6/1 -> re_o/1
  BitBasher5/1 -> im_o/1

== system sysgen_oversample2x_2samples_per_clock/Synthesis/Synthesis/Post_synthesis0 ==
  valid : Inport
  im : Inport  Port=2
  re : Inport  Port=3
  Delay : xbsIndex_r4/Delay  rst=off  infoeditControl=Selection of Reset will increase slice count due to use of real FFs and instead of SRLs  en=off  latency=7  reg_retiming=on  dbl_ovrd=off  block_type=delay
  Delay1 : xbsIndex_r4/Delay  rst=off  infoeditControl=Selection of Reset will increase slice count due to use of real FFs and instead of SRLs  en=off  latency=7  reg_retiming=on  dbl_ovrd=off  block_type=delay
  Delay2 : xbsIndex_r4/Delay  rst=off  infoeditControl=Selection of Reset will increase slice count due to use of real FFs and instead of SRLs  en=off  latency=7  reg_retiming=on  dbl_ovrd=off  block_type=delay
  valid0 : Outport
  im0 : Outport  Port=2
  reo : Outport  Port=3
  wires:
  valid/1 -> Delay/1
  im/1 -> Delay1/1
  re/1 -> Delay2/1
  Delay/1 -> valid0/1
  Delay1/1 -> im0/1
  Delay2/1 -> reo/1

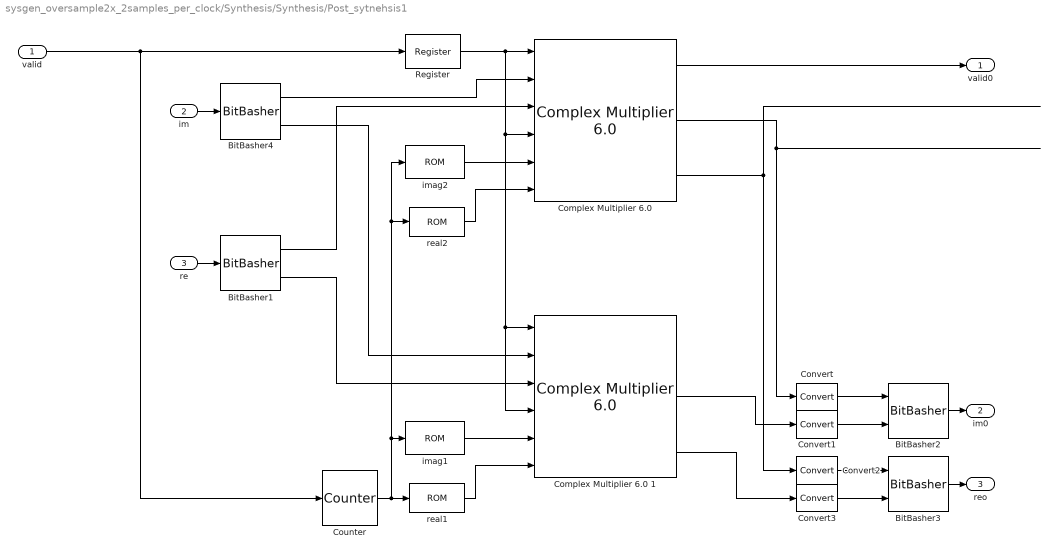
== system sysgen_oversample2x_2samples_per_clock/Synthesis/Synthesis/Post_sytnehsis1 ==
  valid : Inport
  im : Inport  Port=2
  re : Inport  Port=3
  BitBasher1 : xbsIndex_r4/BitBasher  bitexpr=|  display_expr=off  sr_1=hi  arith_type1="Signed  (2's comp)"  bin_pt1=15  sr_2=lo  arith_type2="Signed  (2's comp)"  bin_pt2=15  sr_3=hi  arith_type3=Unsigned  bin_pt3=0  sr_4=4  arith_type4=Unsigned  bin_pt4=0  dbl_ovrd=off  block_type=bitbasher
      | hi = {in[31:16]}
      | lo = {in[15:0]}
  BitBasher2 : xbsIndex_r4/BitBasher  bitexpr=out = {hi, lo}  display_expr=off  sr_1=out  arith_type1=Unsigned  bin_pt1=0  sr_2=hi  arith_type2="Signed  (2's comp)"  bin_pt2=15  sr_3=hi  arith_type3=Unsigned  bin_pt3=0  sr_4=4  arith_type4=Unsigned  bin_pt4=0  dbl_ovrd=off  block_type=bitbasher
  BitBasher3 : xbsIndex_r4/BitBasher  bitexpr=out = {hi, lo}  display_expr=off  sr_1=out  arith_type1=Unsigned  bin_pt1=0  sr_2=hi  arith_type2="Signed  (2's comp)"  bin_pt2=15  sr_3=hi  arith_type3=Unsigned  bin_pt3=0  sr_4=4  arith_type4=Unsigned  bin_pt4=0  dbl_ovrd=off  block_type=bitbasher
  BitBasher4 : xbsIndex_r4/BitBasher  bitexpr=|  display_expr=off  sr_1=hi  arith_type1="Signed  (2's comp)"  bin_pt1=15  sr_2=lo  arith_type2="Signed  (2's comp)"  bin_pt2=15  sr_3=hi  arith_type3=Unsigned  bin_pt3=0  sr_4=4  arith_type4=Unsigned  bin_pt4=0  dbl_ovrd=off  block_type=bitbasher
      | hi = {in[31:16]}
      | lo = {in[15:0]}
  "Complex Multiplier 6.0 " : xbsIndex_r4/Complex Multiplier 6.0   hasatlast=off  hasatuser=off  atuserwidth=1  hasbtlast=off  hasbtuser=off  btuserwidth=1  multtype=Use_Mults  optimizegoal=Resources  flowcontrol=NonBlocking  outputwidth=19  roundmode=Truncate  hasctrltlast=off  hasctrltuser=off  ctrltuserwidth=1  outtlastbehv=Null  latencyconfig=Automatic  minimumlatency=37  aclken=off  aresetn=off  trim_axipin_name=on  simulation_type=hybrid_sim  simulation_model=sysgen:cmpy_v6_0  data_path_portlist={ 's_axis_a_tdata_real', 's_axis_a_tdata_imag', 's_axis_b_tdata_real', 's_axis_b_tdata_imag', 's_axis_ctrl_tdata_rounding_bit', 'm_axis_dout_tdata_real', 'm_axis_dout_tdata_imag' }  aportwidth=63  bportwidth=63  ip_name=Complex Multiplier  ip_version=6.0  dsptool_ready=true  ipcore_usecache=true  ipcore_useipmodelcache=true  ipcore_verbose=false  ipcore_latency_parameter='minimumlatency'  wrapper_available=true  port_translation_map={ 'aclken' => 'en', 'aresetn' => 'rst'}  block_type=cmpy_v6_0
  Complex Multiplier 6.0 1 : xbsIndex_r4/Complex Multiplier 6.0   hasatlast=off  hasatuser=off  atuserwidth=1  hasbtlast=off  hasbtuser=off  btuserwidth=1  multtype=Use_Mults  optimizegoal=Resources  flowcontrol=NonBlocking  outputwidth=19  roundmode=Truncate  hasctrltlast=off  hasctrltuser=off  ctrltuserwidth=1  outtlastbehv=Null  latencyconfig=Automatic  minimumlatency=37  aclken=off  aresetn=off  trim_axipin_name=on  simulation_type=hybrid_sim  simulation_model=sysgen:cmpy_v6_0  data_path_portlist={ 's_axis_a_tdata_real', 's_axis_a_tdata_imag', 's_axis_b_tdata_real', 's_axis_b_tdata_imag', 's_axis_ctrl_tdata_rounding_bit', 'm_axis_dout_tdata_real', 'm_axis_dout_tdata_imag' }  aportwidth=63  bportwidth=63  ip_name=Complex Multiplier  ip_version=6.0  dsptool_ready=true  ipcore_usecache=true  ipcore_useipmodelcache=true  ipcore_verbose=false  ipcore_latency_parameter='minimumlatency'  wrapper_available=true  port_translation_map={ 'aclken' => 'en', 'aresetn' => 'rst'}  block_type=cmpy_v6_0
  Convert{,1..3} (4 alike) : xbsIndex_r4/Convert  gui_display_data_type=Fixed-point  arith_type="Signed  (2's comp)"  n_bits=16  bin_pt=15  float_type=Single  exp_bits=8  fraction_bits=24  quantization=Truncate  overflow=Flag as error  en=off  latency=0  pipeline=off  dbl_ovrd=off  block_type=convert
  Counter : xbsIndex_r4/Counter  cnt_type=Free Running  cnt_to=Inf  operation=Up  start_count=0  cnt_by_val=1  arith_type=Unsigned  n_bits=4  bin_pt=0  load_pin=off  rst=off  en=on  explicit_period=on  period=2  use_behavioral_HDL=off  implementation=Fabric  dbl_ovrd=off  block_type=counter
  Register : xbsIndex_r4/Register  init=0  rst=off  en=off  dbl_ovrd=off  block_type=register
  imag1 : xbsIndex_r4/ROM  depth=16  initVector=imag(exp(j*2*pi*(1:2:31)/32))  distributed_mem=Block RAM  rst=off  init_reg=0  en=off  latency=1  gui_display_data_type=Fixed-point  arith_type="Signed  (2's comp)"  n_bits=18  bin_pt=16  preci_type=Single  exp_width=8  frac_width=24  optimize=Area  use_rpm=on  dbl_ovrd=off  block_type=sprom
  imag2 : xbsIndex_r4/ROM  depth=16  initVector=imag(exp(j*2*pi*(0:2:31)/32))  distributed_mem=Block RAM  rst=off  init_reg=0  en=off  latency=1  gui_display_data_type=Fixed-point  arith_type="Signed  (2's comp)"  n_bits=18  bin_pt=16  preci_type=Single  exp_width=8  frac_width=24  optimize=Area  use_rpm=on  dbl_ovrd=off  block_type=sprom
  real1 : xbsIndex_r4/ROM  depth=16  initVector=real(exp(j*2*pi*(1:2:31)/32))  distributed_mem=Block RAM  rst=off  init_reg=0  en=off  latency=1  gui_display_data_type=Fixed-point  arith_type="Signed  (2's comp)"  n_bits=18  bin_pt=16  preci_type=Single  exp_width=8  frac_width=24  optimize=Area  use_rpm=on  dbl_ovrd=off  block_type=sprom
  real2 : xbsIndex_r4/ROM  depth=16  initVector=real(exp(j*2*pi*(0:2:31)/32))  distributed_mem=Block RAM  rst=off  init_reg=0  en=off  latency=1  gui_display_data_type=Fixed-point  arith_type="Signed  (2's comp)"  n_bits=18  bin_pt=16  preci_type=Single  exp_width=8  frac_width=24  optimize=Area  use_rpm=on  dbl_ovrd=off  block_type=sprom
  valid0 : Outport
  im0 : Outport  Port=2
  reo : Outport  Port=3
  wires:
  im/1 -> BitBasher4/1
  re/1 -> BitBasher1/1
  real2/1 -> "Complex Multiplier 6.0 "/6
  imag2/1 -> "Complex Multiplier 6.0 "/5
  real1/1 -> Complex Multiplier 6.0 1/6
  imag1/1 -> Complex Multiplier 6.0 1/5
  Counter/1 -> imag2/1, real2/1, imag1/1, real1/1
  BitBasher2/1 -> im0/1
  BitBasher3/1 -> reo/1
  valid/1 -> Register/1, Counter/1
  Convert/1 -> BitBasher2/1
  Convert2/1 -> BitBasher3/1
  Convert3/1 -> BitBasher3/2
  Register/1 -> "Complex Multiplier 6.0 "/4, Complex Multiplier 6.0 1/1, Complex Multiplier 6.0 1/4, "Complex Multiplier 6.0 "/1
  "Complex Multiplier 6.0 "/1 -> valid0/1
  Convert1/1 -> BitBasher2/2
  Complex Multiplier 6.0 1/2 -> Convert1/1
  Complex Multiplier 6.0 1/3 -> Convert3/1
  "Complex Multiplier 6.0 "/3 -> Convert2/1
  "Complex Multiplier 6.0 "/2 -> Convert/1
  BitBasher4/1 -> "Complex Multiplier 6.0 "/2
  BitBasher1/1 -> "Complex Multiplier 6.0 "/3
  BitBasher1/2 -> Complex Multiplier 6.0 1/3
  BitBasher4/2 -> Complex Multiplier 6.0 1/2
